simulink model "Taller6_Ejercicio6_4"  (R2024a)
settings: Solver=VariableStepAuto  StartTime=0.0  StopTime=40  RelTol=1e-3
settings Model: Creator=angel  LastModifiedBy=geova

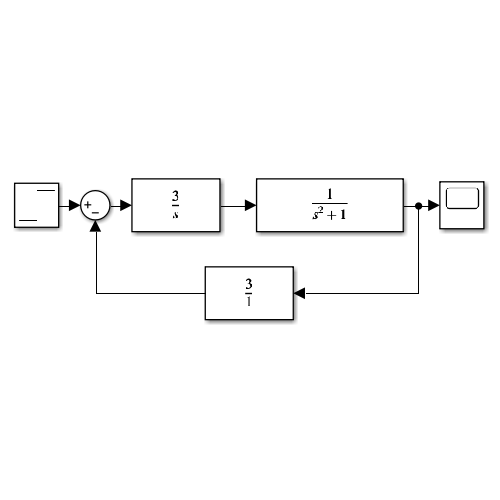
[thumbnail: Simulink's stored preview of the top-level diagram]
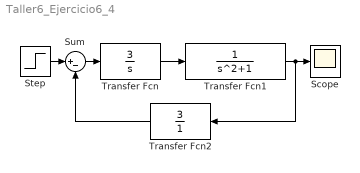
== system Taller6_Ejercicio6_4 ==
  Scope : Scope
  Step : Step  Time=0.025  SampleTime=0.001  ZeroCross=off
  Sum : Sum  Inputs=|+-
  Transfer Fcn : TransferFcn  Numerator=[3]  Denominator=[1 0]
  Transfer Fcn1 : TransferFcn  Denominator=[1 0 1]
  Transfer Fcn2 : TransferFcn  Numerator=3  Denominator=[1]
  wires:
  Step/1 -> Sum/1
  Sum/1 -> Transfer Fcn/1
  Transfer Fcn2/1 -> Sum/2
  Transfer Fcn/1 -> Transfer Fcn1/1
  Transfer Fcn1/1 -> Scope/1, Transfer Fcn2/1
